simulink model "MAS7"  (R2020a)
settings: Solver=ode4  StartTime=start_time  StopTime=stop_time  FixedStep=fixed_step_size  RelTol=1e-3
undefined symbols (not defined in the file): f, J, Kp2, Kp3, Lr, Ls, M, p, Rr, Rs, T_23, T_32, tau2, tau3, taur
libraries: simulink x3
settings Model: Creator=deric  LastModifiedBy=deric

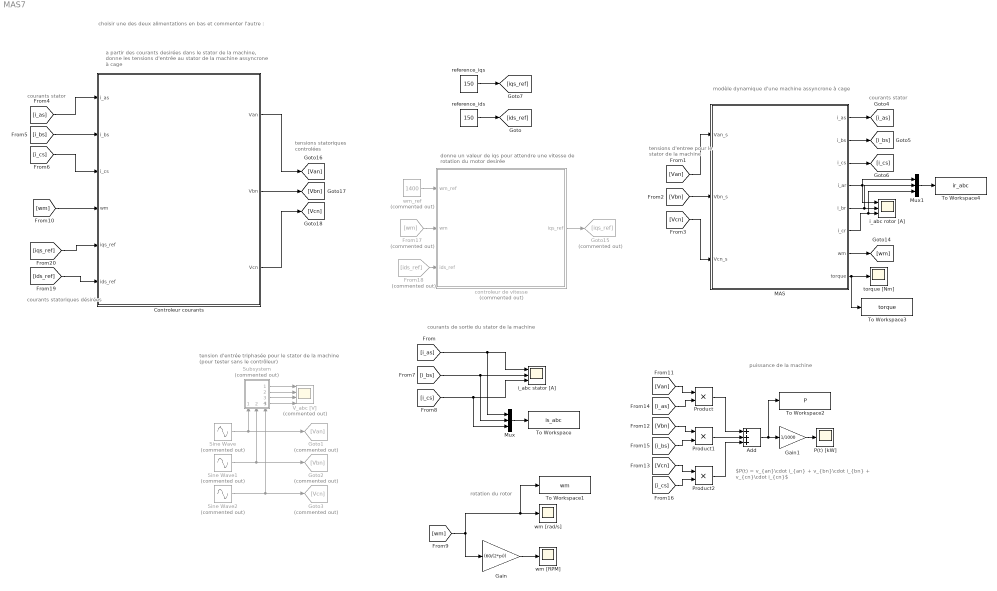
== system MAS7 ==
  note: courants statoriques
      | désirées
  note: courants stator
  note: tensions statoriques
      | controlées
  note: tensions d'entree pour
      | le stator de la machine
  note: courants stator
  note: donne un valeur de iqs pour attendre une vitesse
      | de rotation du motor desirée
  note: choisir une des deux alimentations en bas et commenter l'autre :
  note: a partir des courants desirées dans le stator de la machine,
      | donne les tensions d'entrée au stator de la machine
      | assyncrone à cage
  note: modèle dynamique d'une machine assyncrone à cage
  note: rotation du rotor
  note: courants de sortie du stator de la machine
  note: tension d'entrée triphasée pour le stator de la machine
      | (pour tester sans le contrôleur)
  note: puissance de la machine
  note: $P(t) = v_{an}\cdot i_{an} + v_{bn}\cdot i_{bn} + v_{cn}\cdot i_{cn}$
  Add : Sum  Inputs=+++
  "Controleur courants " : Subsystem
  From17 : From  Commented=on  GotoTag=wm
  From18 : From  Commented=on  GotoTag=ids_ref
  Gain : Gain  Gain=(60/(2*pi))
  Gain1 : Gain  Gain=1/1000
  Goto1 : Goto  Commented=on  GotoTag=Van
  Goto15 : Goto  Commented=on  GotoTag=iqs_ref
  Goto2 : Goto  Commented=on  GotoTag=Vbn
  Goto3 : Goto  Commented=on  GotoTag=Vcn
  MAS : Subsystem
  Mux : Mux  Inputs=3
  Mux1 : Mux  Inputs=3
  P(t) [kW] : Scope
  Product : Product
  Product1 : Product
  Product2 : Product
  Sine Wave : Sin  Commented=on  Amplitude=30  Frequency=300*2*pi  SampleTime=0
  Sine Wave1 : Sin  Commented=on  Amplitude=30  Frequency=300*2*pi  Phase=-2*pi/3  SampleTime=0
  Sine Wave2 : Sin  Commented=on  Amplitude=30  Frequency=300*2*pi  Phase=(2*pi)/3  SampleTime=0
  Subsystem : Subsystem  Commented=on
      settings: PortSchema="{\"entries\":[{\"content\":{\"sides\":[{\"content\":{\"connectorIds\":[]},\"type\":\"ConnectorPlacement.EquallySpacedRectSide\",\"uuid\":\"f85b66a8-0283-4540-940c-33deb3ca5510\"},{\"content\":{\"connectorIds\":[\"Out1\",\"Out2\",\"Out3\",\"Out4\"],\"side\":\"RIGHT\"},\"type\":\"ConnectorPlacement.EquallySpacedRectSide\",\"uuid\":\"e99f7d2c-d092-4cab-bef3-1d0691980dab\"},{\"content\":{\"connectorIds\":[],\"side\":\"TOP\"},\"type\":\"ConnectorPlacement.EquallySpacedRectSide\",\"uuid\":\"dc5a25e5-8be2-48e2-ba29-fa1fa10bdc19\"},{\"content\":{\"connectorIds\":[\"In1\",\"In2\",\"In3\"],\"side\":\"BOTTOM\"},\"type\":\"ConnectorPlacement.EquallySpacedRectSide\",\"uuid\":\"6c390d1e-5fa5-44b0-aac6-b431b338384d\"}]},\"type\":\"ConnectorPlacement.EquallySpacedConnector\",\"uuid\":\"6ae22648-050b-430b-93b5-6047f057b4ba\"}],\"packageUris\":[\"http://schema.mathworks.com/mf0/Connector/19700101\"],\"version\":\"1.0\"}"
  To Workspace : ToWorkspace  VariableName=is_abc  SampleTime=-1
  To Workspace1 : ToWorkspace  VariableName=wm  SampleTime=-1
  To Workspace2 : ToWorkspace  VariableName=P  SampleTime=-1
  To Workspace3 : ToWorkspace  VariableName=torque  SampleTime=-1
  To Workspace4 : ToWorkspace  VariableName=ir_abc  SampleTime=-1
  V_abc [V] : Scope  Commented=on  NumInputPorts=4
  controleur de vitesse : Subsystem  Commented=on
  i_abc rotor [A] : Scope  NumInputPorts=3
  i_abc stator [A] : Scope  NumInputPorts=3
  reference_ids : Constant  Value=150
  reference_iqs : Constant  Value=150
  torque [Nm] : Scope
  wm [RPM] : Scope
  wm [rad/s] : Scope
  wm_ref : Constant  Commented=on  Value=1400
  wires:
  Sine Wave/1 -> Goto1/1, Subsystem/1(In1)
  Sine Wave1/1 -> Goto2/1, Subsystem/2(In2)
  Sine Wave2/1 -> Goto3/1, Subsystem/3(In3)
  [Van] -> MAS/1(Van_s)
  [Vcn] -> MAS/3(Vcn_s)
  MAS/7(wm) -> [wm]
  MAS/5(i_br) -> i_abc rotor [A]/2, Mux1/2
  MAS/4(i_ar) -> i_abc rotor [A]/1, Mux1/1
  MAS/3(i_cs) -> [i_cs]
  MAS/2(i_bs) -> [i_bs]
  MAS/1(i_as) -> [i_as]
  MAS/6(i_cr) -> Mux1/3, i_abc rotor [A]/3
  [i_as] -> "Controleur courants "/1(i_as)
  [i_bs] -> "Controleur courants "/2(i_bs)
  [i_cs] -> "Controleur courants "/3(i_cs)
  [wm] -> "Controleur courants "/4(wm)
  "Controleur courants "/1(Van) -> [Van]
  "Controleur courants "/3(Vcn) -> [Vcn]
  [i_as] -> Mux/1, i_abc stator [A]/1
  [i_bs] -> Mux/2, i_abc stator [A]/2
  [i_cs] -> Mux/3, i_abc stator [A]/3
  [wm] -> To Workspace1/1, wm [rad/s]/1, Gain/1
  Gain/1 -> wm [RPM]/1
  Subsystem/1(Out1) -> V_abc [V]/1
  Subsystem/2(Out2) -> V_abc [V]/2
  Subsystem/3(Out3) -> V_abc [V]/3
  Subsystem/4(Out4) -> V_abc [V]/4
  [Van] -> Product/1
  [i_as] -> Product/2
  [Vbn] -> Product1/1
  [i_bs] -> Product1/2
  [Vcn] -> Product2/1
  [i_cs] -> Product2/2
  Product/1 -> Add/1
  Product1/1 -> Add/2
  Product2/1 -> Add/3
  Add/1 -> To Workspace2/1, Gain1/1
  Gain1/1 -> P(t) [kW]/1
  [Vbn] -> MAS/2(Vbn_s)
  MAS/8(torque) -> torque [Nm]/1, To Workspace3/1
  controleur de vitesse/1(iqs_ref) -> Goto15/1
  "Controleur courants "/2(Vbn) -> [Vbn]
  wm_ref/1 -> controleur de vitesse/1(wm_ref)
  From17/1 -> controleur de vitesse/2(wm)
  Mux/1 -> To Workspace/1
  Mux1/1 -> To Workspace4/1
  From18/1 -> controleur de vitesse/3(ids_ref)
  [ids_ref] -> "Controleur courants "/6(ids_ref)
  [iqs_ref] -> "Controleur courants "/5(iqs_ref)
  reference_iqs/1 -> [iqs_ref]
  reference_ids/1 -> [ids_ref]

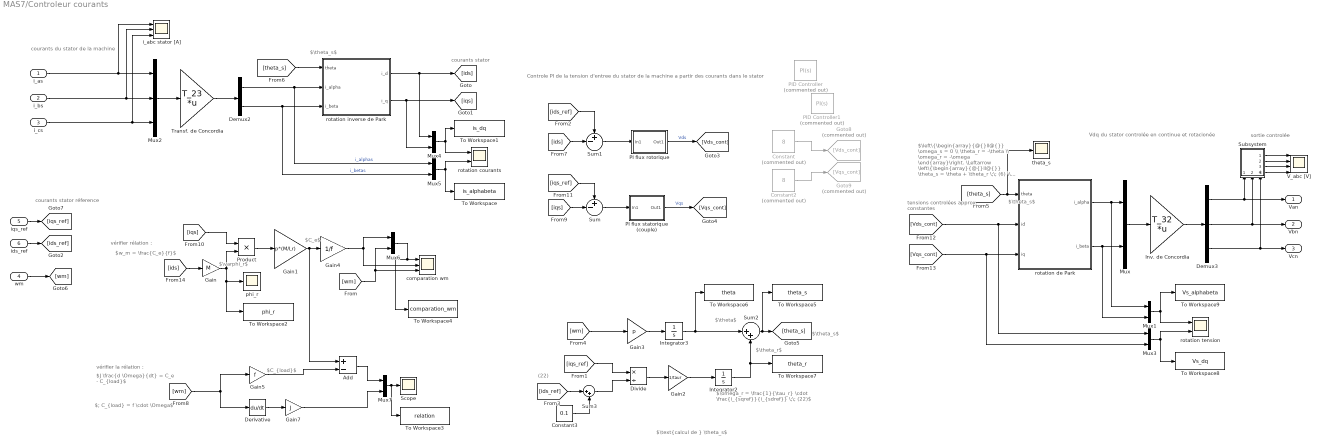
== system MAS7/Controleur courants  ==
  note: tensions controlées
      | approx. constantes
  note: $\text{calcul de } \theta_s$
  note: courants stator réference
  note: courants stator
  note: $; C_{load} = f \cdot \Omega$
  note: $J \frac{d \Omega}{dt} = C_e - C_{load}$
  note: vérifier la rélation :
  note: $C_{load}$
  note: $\varphi_r$
  note: vérifier rélation :
  note: $w_m = \frac{C_e}{f}$
  note: $C_e$
  note: (22)
  note: $\left\{\begin{array}{@{}ll@{}} \omega_s = 0 \\ \theta_r = -\theta \\ \omega_r = -\omega \end{array}\right. \Leftarrow \left\{\begin{array}{@{}ll@{}} \theta_s = \theta + \theta_r \;\; (6) \\ \omega_s = \omega + \omega_r \;\; (7) \\ \theta_s = 0 \;\;(17) \end{array}\right.$
  note: Controle PI de la tension d'entree du stator de la machine a partir des courants dans le stator
  note: courants du stator de la machine
  note: sortie controlée
  note: Vdq du stator controlée en continue et rotacionée
  note: $\theta_s$
  note: $\theta_s$
  note: $\omega_r = \frac{1}{\tau_r} \cdot \frac{i_{sqref}}{i_{sdref}} \;\; (22)$
  note: $\theta$
  note: $\theta_r$
  note: $\theta_s$
  i_as : Inport
  i_bs : Inport  Port=2
  i_cs : Inport  Port=3
  wm : Inport  Port=4
  iqs_ref : Inport  Port=5
  ids_ref : Inport  Port=6
  Add : Sum  Inputs=+-
  Constant : Constant  Commented=on  Value=8  VectorParams1D=off  SampleTime=-1
  Constant2 : Constant  Commented=on  Value=8  VectorParams1D=off  SampleTime=-1
  Constant3 : Constant  Value=0.1
  Demux2 : Demux  Outputs=2
  Demux3 : Demux  Outputs=3
  Derivative : Derivative
  Divide : Product  Inputs=*/
  Gain : Gain  Gain=M
  Gain1 : Gain  Gain=p*(M/Lr)
  Gain2 : Gain  Gain=1/taur
  Gain3 : Gain  Gain=p
  Gain4 : Gain  Gain=1/f
  Gain5 : Gain  Gain=f
  Gain7 : Gain  Gain=J
  Goto8 : Goto  Commented=on  GotoTag=Vds_cont
  Goto9 : Goto  Commented=on  GotoTag=Vqs_cont
  Integrator2 : Integrator
  Integrator3 : Integrator
  Inv. de Concordia : Gain  Gain=T_32  Multiplication=Matrix(K*u)
  Mux{,1,3..7} (7 alike) : Mux  Inputs=2
  Mux2 : Mux  Inputs=3
  PI flux rotorique : Subsystem
  PI flux statorique (couple) : Subsystem
  PID Controller : simulink/Continuous/PID Controller  Commented=on  Controller=PI  Form=Parallel  TimeDomain=Continuous-time  UseExternalTs=off  SampleTime=-1  IntegratorMethod=Forward Euler  FilterMethod=Forward Euler  ControllerParametersSource=internal  P=0  I=0.186222465630192  D=0  UseFilter=on  N=100  TunerSelectOption=Transfer Function Based (PID Tuner App)  InitialConditionSource=internal  InitialConditionForIntegrator=0  InitialConditionForFilter=0  DifferentiatorICPrevScaledInput=0  ExternalReset=none  TrackingMode=off  Kt=1  LimitOutput=off  UpperSaturationLimit=inf  LowerSaturationLimit=-inf  LinearizeAsGain=on  AntiWindupMode=none  Kb=1  POutMin=[]  POutMax=[]  IOutMin=[]  IOutMax=[]  DOutMin=[]  DOutMax=[]  NOutMin=[]  NOutMax=[]  SumOutMin=[]  SumOutMax=[]  SaturationOutMin=[]  SaturationOutMax=[]  PParamMin=[]  PParamMax=[]  IParamMin=[]  IParamMax=[]  DParamMin=[]  DParamMax=[]  NParamMin=[]  NParamMax=[]  KbParamMin=[]  KbParamMax=[]  KtParamMin=[]  KtParamMax=[]  KbOutMin=[]  KbOutMax=[]  KtOutMin=[]  KtOutMax=[]  IntegratorOutMin=[]  IntegratorOutMax=[]  FilterOutMin=[]  FilterOutMax=[]  SumI1OutMin=[]  SumI1OutMax=[]  SumI2OutMin=[]  SumI2OutMax=[]  SumI3OutMin=[]  SumI3OutMax=[]  SumI4OutMin=[]  SumI4OutMax=[]  SumDOutMin=[]  SumDOutMax=[]  DifferentiatorOutMin=[]  DifferentiatorOutMax=[]  FilterDiffOutCoefMin=[]  FilterDiffOutCoefMax=[]  ReciprocalOutMin=[]  ReciprocalOutMax=[]  SumDenOutMin=[]  SumDenOutMax=[]  SumNumOutMin=[]  SumNumOutMax=[]  DivideOutMin=[]  DivideOutMax=[]  UdiffTsProdOutMin=[]  UdiffTsProdOutMax=[]  NTsProdOutMin=[]  NTsProdOutMax=[]  UintegralTsProdOutMin=[]  UintegralTsProdOutMax=[]  UngainTsProdOutMin=[]  UngainTsProdOutMax=[]  IntegratorContinuousStateAttributes=''  IntegratorStateMustResolveToSignalObject=off  IntegratorRTWStateStorageClass=Auto  FilterContinuousStateAttributes=''  FilterStateMustResolveToSignalObject=off  FilterRTWStateStorageClass=Auto  ParallelPVariant=InternalParameters  IdealPVariant=Disabled  IVariant=InternalParameters  DVariant=Disabled  IntegratorVariant=Continuous  SatVariant=Disabled  AWVariant=Passthrough  PCopyVariant=Disabled  TRVariant=Disabled  FdbkBlocksVariant=Forward  IdealPFdbkVariant=Disabled  SatFdbkVariant=Disabled  DerivativeFilterVariant=Disabled  NVariant=Disabled  NCopyVariant=Disabled_SignalSpec  FilterICVariant=Disabled  IntegratorICVariant=InternalICs  ExternalResetVariant=Disabled  TRSumVariant=Passthrough  SumFdbkVariant=Disabled  SumVariant=Sum_PI  TsampFilterVariant=InternalTs  TsampNgainVariant=Passthrough  TsampIntegralVariant=Passthrough
  PID Controller1 : simulink/Continuous/PID Controller  Commented=on  Controller=PI  Form=Parallel  TimeDomain=Continuous-time  UseExternalTs=off  SampleTime=-1  IntegratorMethod=Forward Euler  FilterMethod=Forward Euler  ControllerParametersSource=internal  P=0  I=0.186222465614008  D=0  UseFilter=on  N=100  TunerSelectOption=Transfer Function Based (PID Tuner App)  InitialConditionSource=internal  InitialConditionForIntegrator=0  InitialConditionForFilter=0  DifferentiatorICPrevScaledInput=0  ExternalReset=none  TrackingMode=off  Kt=1  LimitOutput=off  UpperSaturationLimit=inf  LowerSaturationLimit=-inf  LinearizeAsGain=on  AntiWindupMode=none  Kb=1  POutMin=[]  POutMax=[]  IOutMin=[]  IOutMax=[]  DOutMin=[]  DOutMax=[]  NOutMin=[]  NOutMax=[]  SumOutMin=[]  SumOutMax=[]  SaturationOutMin=[]  SaturationOutMax=[]  PParamMin=[]  PParamMax=[]  IParamMin=[]  IParamMax=[]  DParamMin=[]  DParamMax=[]  NParamMin=[]  NParamMax=[]  KbParamMin=[]  KbParamMax=[]  KtParamMin=[]  KtParamMax=[]  KbOutMin=[]  KbOutMax=[]  KtOutMin=[]  KtOutMax=[]  IntegratorOutMin=[]  IntegratorOutMax=[]  FilterOutMin=[]  FilterOutMax=[]  SumI1OutMin=[]  SumI1OutMax=[]  SumI2OutMin=[]  SumI2OutMax=[]  SumI3OutMin=[]  SumI3OutMax=[]  SumI4OutMin=[]  SumI4OutMax=[]  SumDOutMin=[]  SumDOutMax=[]  DifferentiatorOutMin=[]  DifferentiatorOutMax=[]  FilterDiffOutCoefMin=[]  FilterDiffOutCoefMax=[]  ReciprocalOutMin=[]  ReciprocalOutMax=[]  SumDenOutMin=[]  SumDenOutMax=[]  SumNumOutMin=[]  SumNumOutMax=[]  DivideOutMin=[]  DivideOutMax=[]  UdiffTsProdOutMin=[]  UdiffTsProdOutMax=[]  NTsProdOutMin=[]  NTsProdOutMax=[]  UintegralTsProdOutMin=[]  UintegralTsProdOutMax=[]  UngainTsProdOutMin=[]  UngainTsProdOutMax=[]  IntegratorContinuousStateAttributes=''  IntegratorStateMustResolveToSignalObject=off  IntegratorRTWStateStorageClass=Auto  FilterContinuousStateAttributes=''  FilterStateMustResolveToSignalObject=off  FilterRTWStateStorageClass=Auto  ParallelPVariant=InternalParameters  IdealPVariant=Disabled  IVariant=InternalParameters  DVariant=Disabled  IntegratorVariant=Continuous  SatVariant=Disabled  AWVariant=Passthrough  PCopyVariant=Disabled  TRVariant=Disabled  FdbkBlocksVariant=Forward  IdealPFdbkVariant=Disabled  SatFdbkVariant=Disabled  DerivativeFilterVariant=Disabled  NVariant=Disabled  NCopyVariant=Disabled_SignalSpec  FilterICVariant=Disabled  IntegratorICVariant=InternalICs  ExternalResetVariant=Disabled  TRSumVariant=Passthrough  SumFdbkVariant=Disabled  SumVariant=Sum_PI  TsampFilterVariant=InternalTs  TsampNgainVariant=Passthrough  TsampIntegralVariant=Passthrough
  Product : Product
  Scope : Scope
  Subsystem : Subsystem
      settings: PortSchema="{\"entries\":[{\"content\":{\"sides\":[{\"content\":{\"connectorIds\":[]},\"type\":\"ConnectorPlacement.EquallySpacedRectSide\",\"uuid\":\"f85b66a8-0283-4540-940c-33deb3ca5510\"},{\"content\":{\"connectorIds\":[\"Out1\",\"Out2\",\"Out3\",\"Out4\"],\"side\":\"RIGHT\"},\"type\":\"ConnectorPlacement.EquallySpacedRectSide\",\"uuid\":\"e99f7d2c-d092-4cab-bef3-1d0691980dab\"},{\"content\":{\"connectorIds\":[],\"side\":\"TOP\"},\"type\":\"ConnectorPlacement.EquallySpacedRectSide\",\"uuid\":\"dc5a25e5-8be2-48e2-ba29-fa1fa10bdc19\"},{\"content\":{\"connectorIds\":[\"In1\",\"In2\",\"In3\"],\"side\":\"BOTTOM\"},\"type\":\"ConnectorPlacement.EquallySpacedRectSide\",\"uuid\":\"6c390d1e-5fa5-44b0-aac6-b431b338384d\"}]},\"type\":\"ConnectorPlacement.EquallySpacedConnector\",\"uuid\":\"6ae22648-050b-430b-93b5-6047f057b4ba\"}],\"packageUris\":[\"http://schema.mathworks.com/mf0/Connector/19700101\"],\"version\":\"1.0\"}"
  Sum : Sum  Inputs=+-|
  Sum1 : Sum  Inputs=+-|
  Sum2 : Sum  Inputs=|++
  Sum3 : Sum  Inputs=|++
  To Workspace : ToWorkspace  VariableName=is_alphabeta  SampleTime=-1
  To Workspace1 : ToWorkspace  VariableName=is_dq  SampleTime=-1
  To Workspace2 : ToWorkspace  VariableName=phi_r  SampleTime=-1
  To Workspace3 : ToWorkspace  VariableName=relation  SampleTime=-1
  To Workspace4 : ToWorkspace  VariableName=comparation_wm  SampleTime=-1
  To Workspace5 : ToWorkspace  VariableName=theta_s  SampleTime=-1
  To Workspace6 : ToWorkspace  VariableName=theta  SampleTime=-1
  To Workspace7 : ToWorkspace  VariableName=theta_r  SampleTime=-1
  To Workspace8 : ToWorkspace  VariableName=Vs_dq  SampleTime=-1
  To Workspace9 : ToWorkspace  VariableName=Vs_alphabeta  SampleTime=-1
  Transf. de Concordia : Gain  Gain=T_23  Multiplication=Matrix(K*u)
  V_abc [V] : Scope  NumInputPorts=4
  comparation wm : Scope  NumInputPorts=3
  i_abc stator [A] : Scope  NumInputPorts=3
  phi_r : Scope
  "rotation courants " : Scope  NumInputPorts=2
  rotation de Park : MATLAB Function  TreatAsAtomicUnit=on
  rotation inverse de Park : MATLAB Function  TreatAsAtomicUnit=on
  rotation tension : Scope  NumInputPorts=2
  theta_s : Scope
  Van : Outport
  Vbn : Outport  Port=2
  Vcn : Outport  Port=3
  wires:
  Transf. de Concordia/1 -> Demux2/1
  i_cs/1 -> i_abc stator [A]/3, Mux2/3
  i_as/1 -> i_abc stator [A]/1, Mux2/1
  Mux2/1 -> Transf. de Concordia/1
  i_bs/1 -> i_abc stator [A]/2, Mux2/2
  Demux3/2 -> Subsystem/2(In2), Vbn/1
  [Vds_cont] -> Mux3/1, rotation de Park/2(id)
  [Vqs_cont] -> Mux3/2, rotation de Park/3(iq)
  Demux3/3 -> Subsystem/3(In3), Vcn/1
  Demux3/1 -> Subsystem/1(In1), Van/1
  [iqs_ref] -> Sum/1
  [ids_ref] -> Sum1/1
  Constant/1 -> Goto8/1
  Constant2/1 -> Goto9/1
  Demux2/1 -> Mux5/1, rotation inverse de Park/2(i_alpha)  "i_alphas"
  Demux2/2 -> Mux5/2, rotation inverse de Park/3(i_beta)  "i_betas"
  rotation inverse de Park/1(i_d) -> Mux4/1, [ids]
  rotation inverse de Park/2(i_q) -> Mux4/2, [iqs]
  rotation de Park/2(i_beta) -> Mux1/2, Mux/2
  rotation de Park/1(i_alpha) -> Mux1/1, Mux/1
  [ids] -> Sum1/2
  [iqs] -> Sum/2
  Mux/1 -> Inv. de Concordia/1
  Inv. de Concordia/1 -> Demux3/1
  Subsystem/4(Out4) -> V_abc [V]/4
  Subsystem/3(Out3) -> V_abc [V]/3
  Subsystem/2(Out2) -> V_abc [V]/2
  Subsystem/1(Out1) -> V_abc [V]/1
  Mux1/1 -> rotation tension/1, To Workspace9/1
  Mux3/1 -> To Workspace8/1, rotation tension/2
  Mux5/1 -> To Workspace/1, "rotation courants "/2
  Mux4/1 -> To Workspace1/1, "rotation courants "/1
  [theta_s] -> rotation de Park/1(theta), theta_s/1
  [iqs_ref] -> Divide/1
  Divide/1 -> Gain2/1
  Gain2/1 -> Integrator2/1
  Integrator2/1 -> To Workspace7/1, Sum2/2
  Sum2/1 -> To Workspace5/1, [theta_s]
  [theta_s] -> rotation inverse de Park/1(theta)
  [wm] -> Gain3/1
  Gain3/1 -> Integrator3/1
  Integrator3/1 -> To Workspace6/1, Sum2/1
  [ids_ref] -> Sum3/1
  Sum3/1 -> Divide/2
  Constant3/1 -> Sum3/2
  [ids] -> Gain/1
  Gain/1 -> phi_r/1, To Workspace2/1, Product/2
  [iqs] -> Product/1
  Product/1 -> Gain1/1
  Gain1/1 -> Add/1, Gain4/1
  [wm] -> Mux6/2, comparation wm/3
  Mux6/1 -> comparation wm/1, To Workspace4/1
  Gain4/1 -> Mux6/1, comparation wm/2
  [wm] -> Derivative/1, Gain5/1
  Derivative/1 -> Gain7/1
  Add/1 -> Mux7/1
  Gain7/1 -> Mux7/2
  Mux7/1 -> To Workspace3/1, Scope/1
  Gain5/1 -> Add/2
  wm/1 -> [wm]
  ids_ref/1 -> [ids_ref]
  iqs_ref/1 -> [iqs_ref]
  Sum1/1 -> PI flux rotorique/1(In1)
  PI flux rotorique/1(Out1) -> [Vds_cont]  "Vds"
  Sum/1 -> PI flux statorique (couple)/1(In1)
  PI flux statorique (couple)/1(Out1) -> [Vqs_cont]  "Vqs"

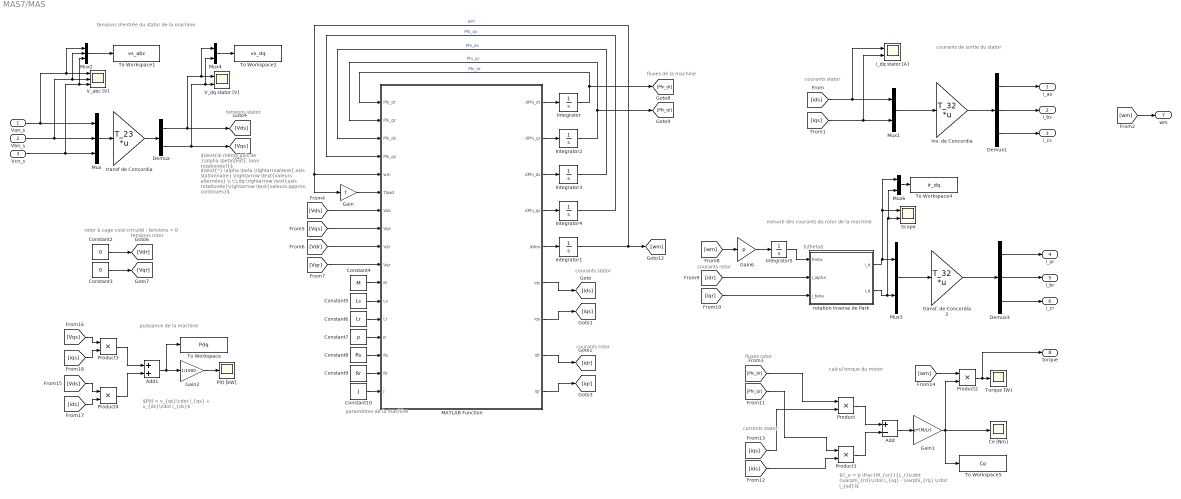
== system MAS7/MAS ==
  note: $\text{*} \alpha \beta \rightarrow\text{ axis stationnaire} \rightarrow \text{valeurs alternées} \\ \;\;dq \rightarrow \text{axis rotationée}\rightarrow \text{valeurs approx. continues}$
  note: $\text{le même axis de }\alpha \beta\text{, (non rotationée)}$
  note: paramètres de
      | la machine
  note: tensions rotor
  note: tensions stator
  note: courants stator
  note: currents stator
  note: fluxes rotor
  note: courants rotor
  note: courants stator
  note: fluxes de la machine
  note: calcul torque du motor
  note: courants de sortie du stator
  note: mesure des courants du rotor de la machine
  note: rotor à cage cout-circuité : tensions = 0
  note: tensions d'entrée du stator de la machine
  note: $C_e = p \frac{M_{sr}}{L_r}\cdot (\varphi_{rd}\cdot i_{sq} - \varphi_{rq} \cdot i_{sd})$
  note: $\theta$
  note: courants rotor
  note: $P(t) = v_{qs}\cdot i_{qs} + v_{ds}\cdot i_{ds}$
  note: puissance de la machine
  Van_s : Inport
  Vbn_s : Inport  Port=2
  Vcn_s : Inport  Port=3
  Add : Sum  Inputs=+-
  Add1 : Sum
  Ce [Nm] : Scope
  Constant10 : Constant  Value=J
  Constant2 : Constant  Value=0
  Constant3 : Constant  Value=0
  Constant4 : Constant  Value=M
  Constant5 : Constant  Value=Ls
  Constant6 : Constant  Value=Lr
  Constant7 : Constant  Value=p
  Constant8 : Constant  Value=Rs
  Constant9 : Constant  Value=Rr
  Demux : Demux  Outputs=2
  Demux1 : Demux  Outputs=3
  Demux3 : Demux  Outputs=3
  Gain : Gain  Gain=f
  Gain1 : Gain  Gain=p*(M/Lr)
  Gain2 : Gain  Gain=1/1000
  Gain6 : Gain  Gain=p
  Integrator{,1..5} (6 alike) : Integrator
  MATLAB Function : MATLAB Function  TreatAsAtomicUnit=on
  Mux : Mux  Inputs=3
  Mux{1,3..4,6} (4 alike) : Mux  Inputs=2
  Mux2 : Mux  Inputs=3
  P(t) [kW] : Scope
  Product{,1..4} (5 alike) : Product
  Scope : Scope  NumInputPorts=2
  To Workspace : ToWorkspace  VariableName=Pdq  SampleTime=-1
  To Workspace1 : ToWorkspace  VariableName=vs_abc  SampleTime=-1
  To Workspace2 : ToWorkspace  VariableName=vs_dq  SampleTime=-1
  To Workspace4 : ToWorkspace  VariableName=ir_dq  SampleTime=-1
  To Workspace5 : ToWorkspace  VariableName=Ce  SampleTime=-1
  Torque [W] : Scope
  V_abc [V] : Scope  NumInputPorts=3
  V_dq stator [V] : Scope  NumInputPorts=2
  i_dq stator [A] : Scope  NumInputPorts=2
  inv. de Concordia : Gain  Gain=T_32  Multiplication=Matrix(K*u)
  rotation inverse de Park : MATLAB Function  TreatAsAtomicUnit=on
  transf de Concordia : Gain  Gain=T_23  Multiplication=Matrix(K*u)
  transf. de Concordia 2 : Gain  Gain=T_32  Multiplication=Matrix(K*u)
  i_as : Outport
  i_bs : Outport  Port=2
  i_cs : Outport  Port=3
  i_ar : Outport  Port=4
  i_br : Outport  Port=5
  i_cr : Outport  Port=6
  wm : Outport  Port=7
  torque : Outport  Port=8
  wires:
  Constant4/1 -> MATLAB Function/11(M)
  [ids] -> i_dq stator [A]/1, Mux1/1
  Constant6/1 -> MATLAB Function/13(Lr)
  [Vdr] -> MATLAB Function/9(Vdr)
  Mux/1 -> transf de Concordia/1
  MATLAB Function/1(dPhi_dr) -> Integrator/1
  Gain/1 -> MATLAB Function/6(Tload)
  [Vqr] -> MATLAB Function/10(Vqr)
  Integrator1/1 -> [wm], MATLAB Function/5(wm), Gain/1  "wm"
  MATLAB Function/7(iqs) -> [iqs]
  Demux/2 -> [Vqs], Mux4/2, V_dq stator [V]/2
  Demux/1 -> Mux4/1, V_dq stator [V]/1, [Vds]
  Vbn_s/1 -> Mux2/2, V_abc [V]/2, Mux/2
  Constant10/1 -> MATLAB Function/17(J)
  [Vds] -> MATLAB Function/7(Vds)
  Integrator2/1 -> MATLAB Function/2(Phi_qr), [Phi_qr]  "Phi_qr"
  Gain6/1 -> Integrator5/1
  Demux1/3 -> i_cs/1
  MATLAB Function/9(iqr) -> [iqr]
  Demux1/1 -> i_as/1
  MATLAB Function/4(dPhi_qs) -> Integrator4/1
  Integrator4/1 -> MATLAB Function/4(Phi_qs)  "Phi_qs"
  Constant7/1 -> MATLAB Function/14(p)
  rotation inverse de Park/1(i_d) -> Mux6/1, Scope/1, Mux3/1
  Demux1/2 -> i_bs/1
  Mux3/1 -> transf. de Concordia 2/1
  [iqs] -> i_dq stator [A]/2, Mux1/2
  Constant3/1 -> [Vqr]
  Constant8/1 -> MATLAB Function/15(Rs)
  MATLAB Function/6(ids) -> [ids]
  Constant2/1 -> [Vdr]
  MATLAB Function/3(dPhi_ds) -> Integrator3/1
  [iqr] -> rotation inverse de Park/3(i_beta)
  Demux3/3 -> i_cr/1
  transf de Concordia/1 -> Demux/1
  Integrator/1 -> [Phi_dr], MATLAB Function/1(Phi_dr)  "Phi_dr"
  inv. de Concordia/1 -> Demux1/1
  MATLAB Function/8(idr) -> [idr]
  MATLAB Function/5(dWm) -> Integrator1/1
  Constant5/1 -> MATLAB Function/12(Ls)
  Demux3/2 -> i_br/1
  Mux1/1 -> inv. de Concordia/1
  [Vqs] -> MATLAB Function/8(Vqs)
  Constant9/1 -> MATLAB Function/16(Rr)
  Integrator3/1 -> MATLAB Function/3(Phi_ds)  "Phi_ds"
  [wm] -> Gain6/1
  MATLAB Function/2(dPhi_qr) -> Integrator2/1
  transf. de Concordia 2/1 -> Demux3/1
  Demux3/1 -> i_ar/1
  rotation inverse de Park/2(i_q) -> Mux6/2, Scope/2, Mux3/2
  Vcn_s/1 -> Mux2/3, V_abc [V]/3, Mux/3
  [idr] -> rotation inverse de Park/2(i_alpha)
  Integrator5/1 -> rotation inverse de Park/1(theta)
  Van_s/1 -> Mux2/1, V_abc [V]/1, Mux/1
  [wm] -> wm/1
  [Phi_qr] -> Product1/1
  [ids] -> Product1/2
  Product/1 -> Add/1
  [Phi_dr] -> Product/1
  [iqs] -> Product/2
  Product1/1 -> Add/2
  Add/1 -> Gain1/1
  Gain1/1 -> To Workspace5/1, Product2/2, Ce [Nm]/1
  [wm] -> Product2/1
  Product2/1 -> torque/1, Torque [W]/1
  [Vqs] -> Product3/1
  [iqs] -> Product3/2
  [Vds] -> Product4/1
  [ids] -> Product4/2
  Product3/1 -> Add1/1
  Product4/1 -> Add1/2
  Gain2/1 -> P(t) [kW]/1
  Add1/1 -> To Workspace/1, Gain2/1
  Mux2/1 -> To Workspace1/1
  Mux4/1 -> To Workspace2/1
  Mux6/1 -> To Workspace4/1

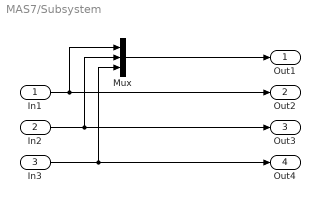
== system MAS7/Subsystem ==
  In1 : Inport
  In2 : Inport  Port=2
  In3 : Inport  Port=3
  Mux : Mux  Inputs=3
  Out1 : Outport
  Out2 : Outport  Port=2
  Out3 : Outport  Port=3
  Out4 : Outport  Port=4
  wires:
  In1/1 -> Mux/1, Out2/1
  In2/1 -> Out3/1, Mux/2
  In3/1 -> Mux/3, Out4/1
  Mux/1 -> Out1/1

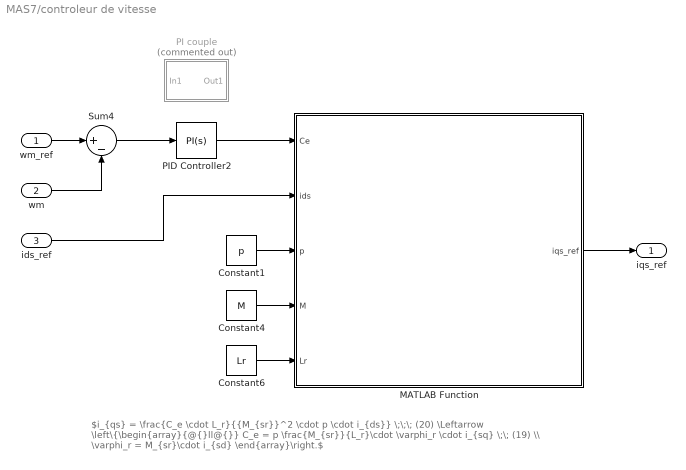
== system MAS7/controleur de vitesse ==
  note: $i_{qs} = \frac{C_e \cdot L_r}{{M_{sr}}^2 \cdot p \cdot i_{ds}} \;\;\; (20) \Leftarrow \left\{\begin{array}{@{}ll@{}} C_e = p \frac{M_{sr}}{L_r}\cdot \varphi_r \cdot i_{sq} \;\; (19) \\ \varphi_r = M_{sr}\cdot i_{sd} \end{array}\right.$
  wm_ref : Inport
  wm : Inport  Port=2
  ids_ref : Inport  Port=3
  Constant1 : Constant  Value=p
  Constant4 : Constant  Value=M
  Constant6 : Constant  Value=Lr
  MATLAB Function : MATLAB Function  TreatAsAtomicUnit=on
  PI couple : Subsystem  Commented=on
  PID Controller2 : simulink/Continuous/PID Controller  Controller=PI  Form=Parallel  TimeDomain=Continuous-time  UseExternalTs=off  SampleTime=-1  IntegratorMethod=Forward Euler  FilterMethod=Forward Euler  ControllerParametersSource=internal  P=0  I=-1  D=0  UseFilter=on  N=100  TunerSelectOption=Transfer Function Based (PID Tuner App)  InitialConditionSource=internal  InitialConditionForIntegrator=0  InitialConditionForFilter=0  DifferentiatorICPrevScaledInput=0  ExternalReset=none  TrackingMode=off  Kt=1  LimitOutput=off  UpperSaturationLimit=inf  LowerSaturationLimit=-inf  LinearizeAsGain=on  AntiWindupMode=none  Kb=1  POutMin=[]  POutMax=[]  IOutMin=[]  IOutMax=[]  DOutMin=[]  DOutMax=[]  NOutMin=[]  NOutMax=[]  SumOutMin=[]  SumOutMax=[]  SaturationOutMin=[]  SaturationOutMax=[]  PParamMin=[]  PParamMax=[]  IParamMin=[]  IParamMax=[]  DParamMin=[]  DParamMax=[]  NParamMin=[]  NParamMax=[]  KbParamMin=[]  KbParamMax=[]  KtParamMin=[]  KtParamMax=[]  KbOutMin=[]  KbOutMax=[]  KtOutMin=[]  KtOutMax=[]  IntegratorOutMin=[]  IntegratorOutMax=[]  FilterOutMin=[]  FilterOutMax=[]  SumI1OutMin=[]  SumI1OutMax=[]  SumI2OutMin=[]  SumI2OutMax=[]  SumI3OutMin=[]  SumI3OutMax=[]  SumI4OutMin=[]  SumI4OutMax=[]  SumDOutMin=[]  SumDOutMax=[]  DifferentiatorOutMin=[]  DifferentiatorOutMax=[]  FilterDiffOutCoefMin=[]  FilterDiffOutCoefMax=[]  ReciprocalOutMin=[]  ReciprocalOutMax=[]  SumDenOutMin=[]  SumDenOutMax=[]  SumNumOutMin=[]  SumNumOutMax=[]  DivideOutMin=[]  DivideOutMax=[]  UdiffTsProdOutMin=[]  UdiffTsProdOutMax=[]  NTsProdOutMin=[]  NTsProdOutMax=[]  UintegralTsProdOutMin=[]  UintegralTsProdOutMax=[]  UngainTsProdOutMin=[]  UngainTsProdOutMax=[]  IntegratorContinuousStateAttributes=''  IntegratorStateMustResolveToSignalObject=off  IntegratorRTWStateStorageClass=Auto  FilterContinuousStateAttributes=''  FilterStateMustResolveToSignalObject=off  FilterRTWStateStorageClass=Auto  ParallelPVariant=InternalParameters  IdealPVariant=Disabled  IVariant=InternalParameters  DVariant=Disabled  IntegratorVariant=Continuous  SatVariant=Disabled  AWVariant=Passthrough  PCopyVariant=Disabled  TRVariant=Disabled  FdbkBlocksVariant=Forward  IdealPFdbkVariant=Disabled  SatFdbkVariant=Disabled  DerivativeFilterVariant=Disabled  NVariant=Disabled  NCopyVariant=Disabled_SignalSpec  FilterICVariant=Disabled  IntegratorICVariant=InternalICs  ExternalResetVariant=Disabled  TRSumVariant=Passthrough  SumFdbkVariant=Disabled  SumVariant=Sum_PI  TsampFilterVariant=InternalTs  TsampNgainVariant=Passthrough  TsampIntegralVariant=Passthrough
  Sum4 : Sum  Inputs=|+-
  iqs_ref : Outport
  wires:
  Constant1/1 -> MATLAB Function/3(p)
  wm/1 -> Sum4/2
  MATLAB Function/1(iqs_ref) -> iqs_ref/1
  Constant6/1 -> MATLAB Function/5(Lr)
  PID Controller2/1 -> MATLAB Function/1(Ce)
  Sum4/1 -> PID Controller2/1
  Constant4/1 -> MATLAB Function/4(M)
  wm_ref/1 -> Sum4/1
  ids_ref/1 -> MATLAB Function/2(ids)

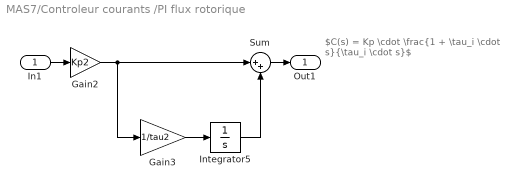
== system MAS7/Controleur courants /PI flux rotorique ==
  note: $C(s) = Kp \cdot \frac{1 + \tau_i \cdot s}{\tau_i \cdot s}$
  In1 : Inport
  Gain2 : Gain  Gain=Kp2
  Gain3 : Gain  Gain=1/tau2
  Integrator5 : Integrator
  Sum : Sum  Inputs=|++
  Out1 : Outport
  wires:
  Gain2/1 -> Sum/1, Gain3/1
  Integrator5/1 -> Sum/2
  Gain3/1 -> Integrator5/1
  In1/1 -> Gain2/1
  Sum/1 -> Out1/1

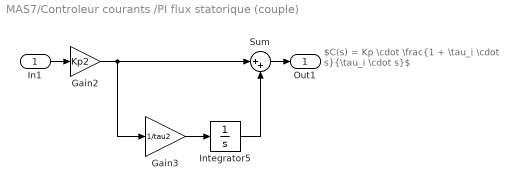
== system MAS7/Controleur courants /PI flux statorique (couple) ==
  note: $C(s) = Kp \cdot \frac{1 + \tau_i \cdot s}{\tau_i \cdot s}$
  In1 : Inport
  Gain2 : Gain  Gain=Kp2
  Gain3 : Gain  Gain=1/tau2
  Integrator5 : Integrator
  Sum : Sum  Inputs=|++
  Out1 : Outport
  wires:
  Gain2/1 -> Sum/1, Gain3/1
  Integrator5/1 -> Sum/2
  Gain3/1 -> Integrator5/1
  In1/1 -> Gain2/1
  Sum/1 -> Out1/1

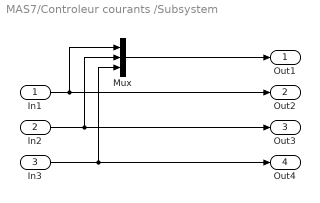
== system MAS7/Controleur courants /Subsystem ==
  In1 : Inport
  In2 : Inport  Port=2
  In3 : Inport  Port=3
  Mux : Mux  Inputs=3
  Out1 : Outport
  Out2 : Outport  Port=2
  Out3 : Outport  Port=3
  Out4 : Outport  Port=4
  wires:
  In1/1 -> Mux/1, Out2/1
  In2/1 -> Out3/1, Mux/2
  In3/1 -> Mux/3, Out4/1
  Mux/1 -> Out1/1

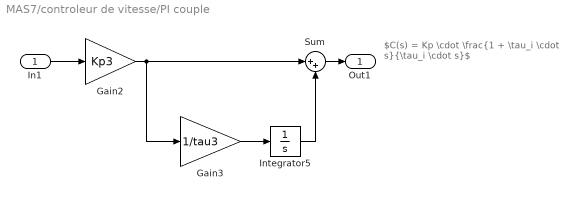
== system MAS7/controleur de vitesse/PI couple ==
  note: $C(s) = Kp \cdot \frac{1 + \tau_i \cdot s}{\tau_i \cdot s}$
  In1 : Inport
  Gain2 : Gain  Gain=Kp3
  Gain3 : Gain  Gain=1/tau3
  Integrator5 : Integrator
  Sum : Sum  Inputs=|++
  Out1 : Outport
  wires:
  Gain2/1 -> Sum/1, Gain3/1
  Integrator5/1 -> Sum/2
  Gain3/1 -> Integrator5/1
  In1/1 -> Gain2/1
  Sum/1 -> Out1/1

== matlab function MAS7/MAS/rotation inverse de Park ==
  data: theta input; i_d output; i_alpha input; i_beta input; i_q output
function [i_d,i_q] = P_mtheta(theta, i_alpha, i_beta)
% P_theta Réalise la transformation inverse de Park.
%
% Cette fonction applique la transformation inverse de Park pour convertir les courants
% de l'axe alpha-bêta vers l'axe d-q (direct-quadrature).
% La transformation de Park est couramment utilisée dans le contrôle des moteurs AC
% et les onduleurs de puissance.
%
% Arguments :
%   theta (float): L'angle de rotation en radians.
%   i_d (float): Composant du courant sur l'axe alpha. 
%   i_q (float): Composant du courant sur l'axe bêta. 
%
% Retour :
%   i_alpha (float): Composant du courant sur l'axe direct après transformation.
%   i_beta (float): Composant du courant sur l'axe en quadrature après transformation.


P_mtheta = [cos(theta) sin(theta); -sin(theta) cos(theta)];
i_alphabeta = [i_alpha, i_beta]';

i_dq = P_mtheta*i_alphabeta; 

i_d = i_dq(1);
i_q = i_dq(2);

== matlab function MAS7/Controleur courants /rotation de Park ==
  data: theta input; i_alpha output; id input; iq input; i_beta output
function [i_alpha,i_beta] = P_theta(theta, id, iq)
% P_theta Réalise la transformation de Park.
%
% Cette fonction applique la transformation de Park pour convertir 
% les courants de l'axe d-q (direct-quadrature) vers l'axe alpha-bêta.
% La transformation de Park est couramment utilisée dans le contrôle des 
% moteurs AC et les onduleurs de puissance.
%
% Arguments :
%   theta (float): L'angle de rotation en radians.
%   id (float): Composant du courant sur l'axe direct.
%   iq (float): Composant du courant sur l'axe en quadrature.
%
% Retour :
%   i_alpha (float): Composant du courant sur l'axe alpha après transformation.
%   i_beta (float): Composant du courant sur l'axe bêta après transformation.

P_theta = [cos(theta) -sin(theta); sin(theta) cos(theta)];
i_dq = [id, iq]';

i_alphabeta = P_theta*i_dq; 

i_alpha = i_alphabeta(1);
i_beta = i_alphabeta(2);

== matlab function MAS7/MAS/MATLAB Function ==
  data: dPhi_dr output; dPhi_qr output; Phi_dr input; dPhi_ds output; dPhi_qs output; dWm output; Phi_qr input; Phi_ds input; Phi_qs input; wm input; Tload input; Vds input; Vqs input; Vdr input; Vqr input; M input; Ls input; Lr input; p input; ids output; iqs output; idr output; iqr output; Rs input; Rr input; J input
 function [dPhi_dr,dPhi_qr,dPhi_ds,dPhi_qs,dWm,ids,iqs,idr,iqr] = dynamique_machine(Phi_dr,Phi_qr,Phi_ds,Phi_qs,wm,Tload,Vds,Vqs,Vdr,Vqr,M,Ls,Lr,p,Rs,Rr,J)

% dPhi Calcul de la dérivée du flux de liaison magnétique, de la dérivée de la vitesse mécanique de l'arbre et du courant dans une machine asynchrone
% 
% Inputs:
%   Phis  : Vecteur des flux de liaison magnétiques
%   wm    : Vitesse mécanique de l'arbre
%   V     : Vecteur des tensions 
%   Tload : Couple de charge
%   ML    : Matrice d'inductance de la machine
%   p     : Nombre de pôles de la machine
%   R     : Matrice de résistance diagonale pour les enroulements stator et rotor
%
% Outputs:
%   dPhis : Vecteur de la dérivée du flux de liaison magnétique
%   dWm   : Dérivée de la vitesse mécanique de l'arbre
%   I     : Vecteur des courants 

% Initialisation de la vitesse angulaire statorique 
%à zéro (référentiel tournant)
ws = 0;

% Calcul de la vitesse angulaire rotorique à partir 
%de la vitesse mécanique
wr = -p*wm; % wm = W mécanique

% Calcul des courants à partir des flux de liaison magnétiques 
%et de la matrice d'inductance 
Phis = [Phi_ds,Phi_qs,Phi_dr,Phi_qr];
ML = [Ls 0 M 0; 0 Ls 0 M; M 0 Lr 0; 0 M 0 Lr];
LM=inv(ML);

I=LM*Phis';

ids=I(1);
iqs=I(2);
idr=I(3);
iqr=I(4);


% Calcul de la dérivée des flux de liaison magnétiques 
dPhi_ds = Vds - Rs*ids + ws*Phi_qs;
dPhi_qs = Vqs - Rs*iqs - ws*Phi_ds;
dPhi_dr = Vdr - Rr*idr + wr*Phi_qr;
dPhi_qr = Vqr - Rr*iqr - wr*Phi_dr;

% calcule le couple électromagnétique
%Tem = p*(Phi_ds*iqs - Phi_qs*ids);
Tem = p*(M/Lr)*(Phi_dr*iqs - Phi_qr*ids);

% Calcul de la dérivée de la vitesse mécanique
dWm = (1/J)*(Tem - Tload);

== matlab function MAS7/controleur de vitesse/MATLAB Function ==
  data: Ce input; iqs_ref output; ids input; p input; M input; Lr input
function iqs_ref  = couplage(Ce,ids,p,M,Lr)

iqs_ref = (Ce*Lr)/((M^2)*p*ids);

== matlab function MAS7/Controleur courants /rotation inverse de Park ==
  data: theta input; i_d output; i_alpha input; i_beta input; i_q output
function [i_d,i_q] = P_mtheta(theta, i_alpha, i_beta)
% P_theta Réalise la transformation inverse de Park.
%
% Cette fonction applique la transformation inverse de Park pour convertir les courants
% de l'axe alpha-bêta vers l'axe d-q (direct-quadrature).
% La transformation de Park est couramment utilisée dans le contrôle des moteurs AC
% et les onduleurs de puissance.
%
% Arguments :
%   theta (float): L'angle de rotation en radians.
%   i_d (float): Composant du courant sur l'axe alpha. 
%   i_q (float): Composant du courant sur l'axe bêta. 
%
% Retour :
%   i_alpha (float): Composant du courant sur l'axe direct après transformation.
%   i_beta (float): Composant du courant sur l'axe en quadrature après transformation.


P_mtheta = [cos(theta) sin(theta); -sin(theta) cos(theta)];
i_alphabeta = [i_alpha, i_beta]';

i_dq = P_mtheta*i_alphabeta; 

i_d = i_dq(1);
i_q = i_dq(2);
